simulink model "AGTF30_eng"  (R2023b)
settings: Solver=FixedStepDiscrete  StartTime=0.0  StopTime=10.0  FixedStep=0.015  RelTol=1e-3  SampleTimeConstraint=STIndependent  EnableMultiTasking=on
model workspace: external: MAT-File (data not in the file)
values from neighbouring files (symbols this model uses):
  MWS = setup_initialize(MWS,startPt,SSsolverSP)    [Setup_Simulation.m]    (also in run_AGTF30e_script.m = Setup_Simulation(inputMethod,MWS.In,filename,Mdl,SSsolverSP))
undefined symbols (not defined in the file or in its folder): stripchar_TMATS
libraries: Lib_Turbo_StaticCalc_TMATS x6, Lib_Turbo_Compressor_TMATS x3, Lib_Turbo_TurbineNPSS_TMATS x2, Lib_Turbo_Shaft_TMATS x2, Lib_Turbo_Ambient_TMATS x1, Lib_Turbo_Nozzle_TMATS x1, Lib_Turbo_NozzleVar_TMATS x1, Lib_Turbo_Burner_TMATS x1, Lib_Turbo_GearBox_TMATS x1, Lib_Turbo_Inlet_TMATS x1, Lib_Turbo_Splitter_TMATS x1, Lib_Turbo_Valve_TMATS x1
(part 2 of 2)

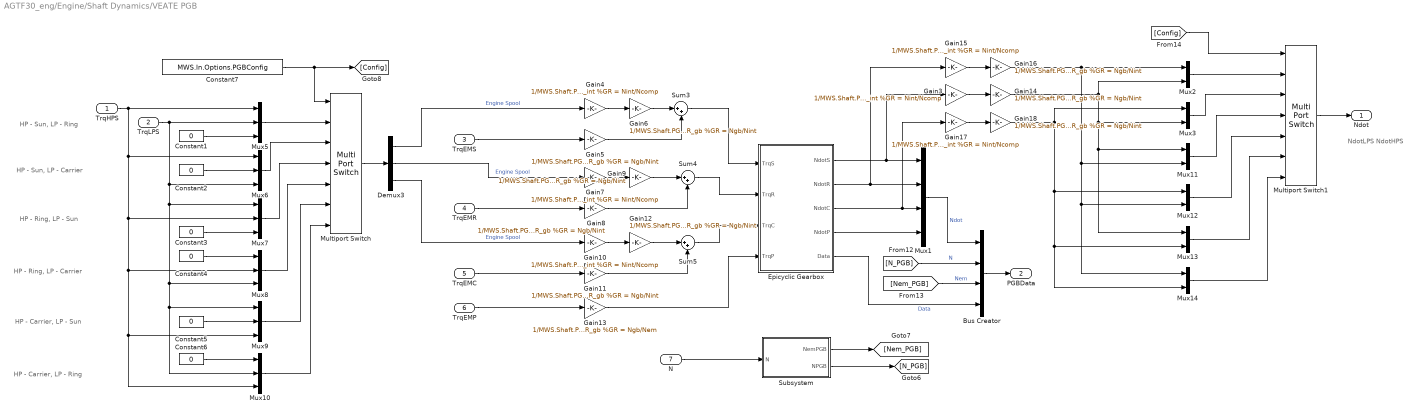
== system AGTF30_eng/Engine/Shaft Dynamics/VEATE PGB ==
  note: NdotLPS
      | NdotHPS
  note: HP - Sun, LP - Ring
  note: HP - Sun, LP - Carrier
  note: HP - Ring, LP - Sun
  note: HP - Ring, LP - Carrier
  note: HP - Carrier, LP - Sun
  note: HP - Carrier, LP - Ring
  TrqHPS : Inport
  TrqLPS : Inport  Port=2
  TrqEMS : Inport  Port=3
  TrqEMR : Inport  Port=4
  TrqEMC : Inport  Port=5
  TrqEMP : Inport  Port=6
  N : Inport  Port=7
  Bus Creator : BusCreator  Inputs=4
  Constant{1..6} (6 alike) : Constant  Value=0
  Constant7 : Constant  Value=MWS.In.Options.PGBConfig
  Demux3 : Demux  Outputs=3
  Epicyclic Gearbox : Subsystem  mask(Epicyclic Gearbox){nP_M=MWS.Shaft.PGB.Planet.nP, mP_M=MWS.Shaft.PGB.Planet.mP, rS_M=MWS.Shaft.PGB.Sun.r, rR_M=MWS.Shaft.PGB.Ring.r, JS_M=MWS.Shaft.PGB.Sun.J, JR_M=MWS.Shaft.PGB.Ring.J, JC_M=MWS.Shaft.PGB.Carrier.J, JP_M=MWS.Shaft.PGB.Planet.J}
      mask prompts: nP_M "nP_M - number of planets"; mP_M "mP_M - mass of each planet gear"; rS_M "rS_M - radius of the sun gear, ft"; rR_M "rR_M - radius of the ring gear, ft"; JS_M "JS_M - inertia of the sun gear, slug-ft^2"; JR_M "JR_M - inertia of the ring gear, slug-ft^2"; JC_M "JC_M - inertia of the carrier, slug-ft^2"; JP_M "JP_M - inertia of each planet gear, slug-ft^2"
      mask help:
      | This block models the dynamics of an epicyclic gearbox. The gearbox is made up of 3 primary components: the sun gear, the ring gear, and the carrier. The carrier is connected through axles to several planet gears that spin between the sun gear and the ring gear. Torque can be input on the sun gear (TrqS), ring gear (TrqR), carrier (TrqC), or planet gears (TrqP). The torques should be supplied in units of ft-lbf. TrqP is assumed to be applied to each planet gear. All (+) torques are prescribed to be in the same direction. This block computes the acceleration in rpm/s of each component (sun gear, ring gear, carrier, and planet gear) which can be integrated outside of the block to obtain the component speeds in rpm. The user should take care to properly intialize the speeds of the components such that the velocity of the gears at their interfaces match. In other words the following relations should be satisfied:
      |
      | rS*NC - rP*NP = rS*NS
      | rR*NC + rP*NP = rR*NR
      |
      | Given the speed of 2 of the components, the other 2 speeds can be computed. The block also provides supplemental data through the output 'Data'. This includes the forces acting at each gear interface and the effective inertia of each component. The effective inertia is defined here as the inertia experienced by the component, which accounts for the reflected inertia of the rest of the mechanical system. Also included are coefficients that describe how applying torque with each component translates to torque applied to the other components. The torque coefficients can be used together with compoent speed information to compute the impact of the gearbox relative to power injection/extraction on each component. The final parameter of the 'Data" structure is an error term that provides some evidence for confidence in the blocks calculations. The NdotErr parameter is a 4 element array that gives the difference in component accelerations calculated 2 different ways. The 4 elements of the array correspond to the sun gear, ring gear, carrier, and planet gear. For clarity, the contents of the 'Data" output are shown below:
      |
      | fsp: force in lbf acting at the sun gear and planet gear interface
      | fpr: force in lbf acting at the planet gear and ring gear interface
      | fpc: force in lbf acting at the axle connecting the planet gear to the carrier
      | JSeff: effective inertia in slug-ft^2 as seen by the sun gear
      | JReff: effective inertia in slug-ft^2 as seen by the ring gear
      | JCeff: effective inertia in slug-ft^2 as seen by the carrier
      | CTrqSR: torque coefficient relating TrqR to the torque it results in on the sun gear
      | CTrqSC: torque coefficient relating TrqC to the torque it results in on the sun gear
      | CTrqSP: torque coefficient relating TrqP to the torque it results in on the sun gear
      | CTrqRS: torque coefficient relating TrqS to the torque it results in on the ring gear
      | CTrqRC: torque coefficient relating TrqC to the torque it results in on the ring gear
      | CTrqRP: torque coefficient relating TrqP to the torque it results in on the ring gear
      | CTrqCS: torque coefficient relating TrqS to the torque it results in on the carrier
      | CTrqCR: torque coefficient relating TrqR to the torque it results in on the carrier
      | CTrqCP: torque coefficient relating TrqP to the torque it results in on the carrier
      | NdotErr: error of the component (sun gear, ring gear, carrier, planet gear) acceleratons calculated 2 separate ways.
      mask init:
      | % Planet Radius
      | rP_I = 0.5*(rR_M-rS_M);
      | % Tier 1 Simplifiers
      | lam_I = 1/(mP_M*(rS_M+rP_I));
      | zeta_I = (1/JC_M)*nP_M*(rS_M+rP_I);
      | theta_I = rP_I^2/JP_M + nP_M*rS_M^2/JS_M;
      | xi_I = rP_I^2/JP_M + nP_M*rR_M^2/JR_M;
      | % Tier 2 Simplifiers
      | phi_I = -theta_I - rP_I^2/JP_M;
      | % Tier 3 Simplifiers
      | sig_I = (1/phi_I)*(rS_M*zeta_I + theta_I*(1+zeta_I/lam_I));
      | eta_I = (1/phi_I)*(1/JC_M)*(rS_M+theta_I/lam_I);
      | alpha_I = -(rS_M/JS_M)*(1/phi_I)*(rP_I^2/JP_M+xi_I);
      | nu_I = (rP_I/JP_M)*(-(1/phi_I)*(rP_I^2/JP_M)+(-xi_I/phi_I-1));
      | % Tier 4 Simplifiers
      | gam_I = -(rP_I^2/JP_M)*(sig_I+(1+zeta_I/lam_I)) - sig_I*xi_I + rR_M*zeta_I;
      | kappa_I = sig_I + (1+zeta_I/lam_I);
      | beta_I = (rP_I^2/JP_M)*(eta_I+(1/lam_I)*(1/JC_M)) + eta_I*xi_I - rR_M/JC_M;
      | % Effective Inertias
      | JSeff_I = JS_M/(1-nP_M*rS_M*(kappa_I*alpha_I/gam_I-(1/phi_I)*rS_M/JS_M));
      | JReff_I = JR_M/(1+nP_M*(sig_I/gam_I)*(rR_M^2/JR_M));
      | JCeff_I = JC_M/(1+nP_M*(rS_M+rP_I)*beta_I/gam_I);
      | % Effective Torque Coefficients
      | CTrqSR_I = -(nP_M*rS_M*(kappa_I/gam_I)*rR_M/JR_M)/(1-nP_M*rS_M*(kappa_I*alpha_I/gam_I-(1/phi_I)*rS_M/JS_M));
      | CTrqSC_I = -(nP_M*rS_M*(kappa_I*beta_I/gam_I+eta_I+(1/lam_I)*(1/JC_M)))/(1-nP_M*rS_M*(kappa_I*alpha_I/gam_I-(1/phi_I)*rS_M/JS_M));
      | CTrqSP_I = -(nP_M*rS_M*(kappa_I*nu_I/gam_I-(1/phi_I)*(rP_I/JP_M)))/(1-nP_M*rS_M*(kappa_I*alpha_I/gam_I-(1/phi_I)*rS_M/JS_M));
      | CTrqRS_I = (nP_M*rR_M*(sig_I*alpha_I/gam_I-(1/phi_I)*rS_M/JS_M))/(1+nP_M*(sig_I/gam_I)*(rR_M^2/JR_M));
      | CTrqRC_I = (nP_M*rR_M*(sig_I*beta_I/gam_I+eta_I))/(1+nP_M*(sig_I/gam_I)*(rR_M^2/JR_M));
      | CTrqRP_I = (nP_M*rR_M*(sig_I*nu_I/gam_I-(1/phi_I)*(rP_I/JP_M)))/(1+nP_M*(sig_I/gam_I)*(rR_M^2/JR_M));
      | CTrqCS_I = (nP_M*(rS_M+rP_I)*alpha_I)/(gam_I+nP_M*(rS_M+rP_I)*beta_I);
      | CTrqCR_I = (nP_M*(rS_M+rP_I)*(rR_M/JR_M))/(gam_I+nP_M*(rS_M+rP_I)*beta_I);
      | CTrqCP_I = (nP_M*(rS_M+rP_I)*nu_I)/(gam_I+nP_M*(rS_M+rP_I)*beta_I);
  Gain10 : Gain  Gain=1/MWS.Shaft.PGB.Carrier.GR_int %GR = Nint/Ncomp
  Gain11 : Gain  Gain=1/MWS.Shaft.PGB.Carrier.GR_gb %GR = Ngb/Nint
  Gain12 : Gain  Gain=1/MWS.Shaft.PGB.Carrier.GR_gb %GR = Ngb/Nint
  Gain13 : Gain  Gain=1/MWS.Shaft.PGB.Planet.GR_gb %GR = Ngb/Nem
  Gain14 : Gain  Gain=1/MWS.Shaft.PGB.Sun.GR_gb %GR = Ngb/Nint
  Gain15 : Gain  Gain=1/MWS.Shaft.PGB.Ring.GR_int %GR = Nint/Ncomp
  Gain16 : Gain  Gain=1/MWS.Shaft.PGB.Ring.GR_gb %GR = Ngb/Nint
  Gain17 : Gain  Gain=1/MWS.Shaft.PGB.Carrier.GR_int %GR = Nint/Ncomp
  Gain18 : Gain  Gain=1/MWS.Shaft.PGB.Carrier.GR_gb %GR = Ngb/Nint
  Gain3 : Gain  Gain=1/MWS.Shaft.PGB.Sun.GR_int %GR = Nint/Ncomp
  Gain4 : Gain  Gain=1/MWS.Shaft.PGB.Sun.GR_int %GR = Nint/Ncomp
  Gain5 : Gain  Gain=1/MWS.Shaft.PGB.Sun.GR_gb %GR = Ngb/Nint
  Gain6 : Gain  Gain=1/MWS.Shaft.PGB.Sun.GR_gb %GR = Ngb/Nint
  Gain7 : Gain  Gain=1/MWS.Shaft.PGB.Ring.GR_int %GR = Nint/Ncomp
  Gain8 : Gain  Gain=1/MWS.Shaft.PGB.Ring.GR_gb %GR = Ngb/Nint
  Gain9 : Gain  Gain=1/MWS.Shaft.PGB.Ring.GR_gb %GR = Ngb/Nint
  Multiport Switch : MultiPortSwitch  Inputs=6  SaturateOnIntegerOverflow=off  InputSameDT=off
  Multiport Switch1 : MultiPortSwitch  Inputs=6  SaturateOnIntegerOverflow=off  InputSameDT=off
  Mux1 : Mux
  Mux{5..10} (6 alike) : Mux  Inputs=3
  Mux{2..3,11..14} (6 alike) : Mux  Inputs=2
  Subsystem : Subsystem
  Sum3 : Sum  Inputs=|++
  Sum4 : Sum  Inputs=|++
  Sum5 : Sum  Inputs=|++
  Ndot : Outport
  PGBData : Outport  Port=2
  wires:
  Constant5/1 -> Mux9/2
  Gain5/1 -> Sum3/2
  Gain14/1 -> Mux13/1, Mux11/1, Mux3/2, Mux2/2
  Constant3/1 -> Mux7/3
  Mux2/1 -> Multiport Switch1/2
  Mux5/1 -> Multiport Switch/2
  Gain4/1 -> Gain6/1
  Epicyclic Gearbox/2(NdotR) -> Gain15/1, Mux1/2
  Gain10/1 -> Gain12/1
  Mux14/1 -> Multiport Switch1/7
  Gain16/1 -> Mux14/1, Mux12/2, Mux11/2, Mux2/1
  Mux11/1 -> Multiport Switch1/4
  Mux13/1 -> Multiport Switch1/6
  Gain18/1 -> Mux14/2, Mux13/2, Mux12/1, Mux3/1
  Constant1/1 -> Mux5/3
  Gain12/1 -> Sum5/1
  [Config] -> Multiport Switch1/1
  Gain6/1 -> Sum3/1
  Constant7/1 -> Multiport Switch/1, [Config]
  Epicyclic Gearbox/3(NdotC) -> Gain17/1, Mux1/3
  Gain9/1 -> Sum4/1
  Mux3/1 -> Multiport Switch1/3
  Constant4/1 -> Mux8/1
  Gain15/1 -> Gain16/1
  Mux12/1 -> Multiport Switch1/5
  Sum3/1 -> Epicyclic Gearbox/1(TrqS)
  Constant6/1 -> Mux10/1
  Mux10/1 -> Multiport Switch/7
  Epicyclic Gearbox/1(NdotS) -> Gain3/1, Mux1/1
  Gain13/1 -> Epicyclic Gearbox/4(TrqP)
  Gain3/1 -> Gain14/1
  Constant2/1 -> Mux6/2
  Gain17/1 -> Gain18/1
  TrqHPS/1 -> Mux10/3, Mux9/3, Mux8/2, Mux7/2, Mux6/1, Mux5/1
  TrqEMP/1 -> Gain13/1
  Demux3/1 -> Gain4/1  "Engine Spool"
  Demux3/3 -> Gain10/1  "Engine Spool"
  Sum4/1 -> Epicyclic Gearbox/2(TrqR)
  Gain8/1 -> Sum4/2
  Mux8/1 -> Multiport Switch/5
  Multiport Switch/1 -> Demux3/1
  Gain11/1 -> Sum5/2
  Sum5/1 -> Epicyclic Gearbox/3(TrqC)
  TrqLPS/1 -> Mux6/3, Mux7/1, Mux8/3, Mux9/1, Mux10/2, Mux5/2
  Gain7/1 -> Gain9/1
  Mux7/1 -> Multiport Switch/4
  Mux6/1 -> Multiport Switch/3
  Demux3/2 -> Gain7/1  "Engine Spool"
  Mux9/1 -> Multiport Switch/6
  TrqEMC/1 -> Gain11/1
  Epicyclic Gearbox/4(NdotP) -> Mux1/4
  Mux1/1 -> Bus Creator/1  "Ndot"
  Multiport Switch1/1 -> Ndot/1
  TrqEMR/1 -> Gain8/1
  TrqEMS/1 -> Gain5/1
  Epicyclic Gearbox/5(Data) -> Bus Creator/4  "Data"
  Bus Creator/1 -> PGBData/1
  [N_PGB] -> Bus Creator/2  "N"
  [Nem_PGB] -> Bus Creator/3  "Nem"
  N/1 -> Subsystem/1(N)
  Subsystem/1(NemPGB) -> [Nem_PGB]
  Subsystem/2(NPGB) -> [N_PGB]

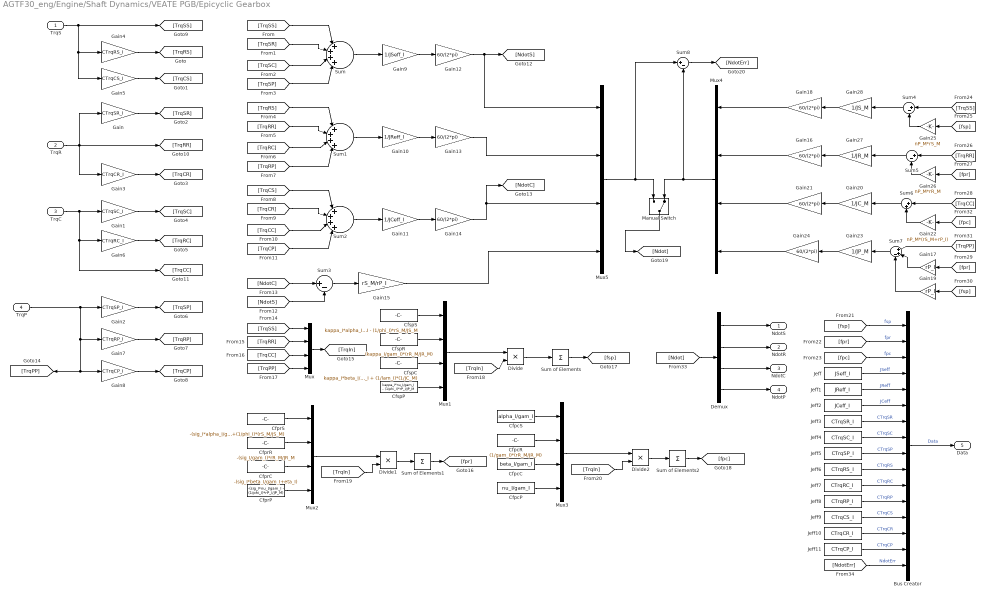
== system AGTF30_eng/Engine/Shaft Dynamics/VEATE PGB/Epicyclic Gearbox ==
  TrqS : Inport
  TrqR : Inport  Port=2
  TrqC : Inport  Port=3
  TrqP : Inport  Port=4
  Bus Creator : BusCreator  Inputs=16
  CfpcC : Constant  Value=beta_I/gam_I
  CfpcP : Constant  Value=nu_I/gam_I
  CfpcR : Constant  Value=(1/gam_I)*(rR_M/JR_M)
  CfpcS : Constant  Value=alpha_I/gam_I
  CfprC : Constant  Value=-(sig_I*beta_I/gam_I+eta_I)
  CfprP : Constant  Value=-(sig_I*nu_I/gam_I - (1/phi_I)*rP_I/JP_M)
  CfprR : Constant  Value=-(sig_I/gam_I)*rR_M/JR_M
  CfprS : Constant  Value=-(sig_I*alpha_I/gam_I)+(1/phi_I)*(rS_M/JS_M)
  CfspC : Constant  Value=kappa_I*beta_I/gam_I + eta_I + (1/lam_I)*(1/JC_M)
  CfspP : Constant  Value=kappa_I*nu_I/gam_I - (1/phi_I)*rP_I/JP_M
  CfspR : Constant  Value=(kappa_I/gam_I)*(rR_M/JR_M)
  CfspS : Constant  Value=kappa_I*alpha_I/gam_I - (1/phi_I)*rS_M/JS_M
  Demux : Demux
  Divide : Product  Inputs=**
  Divide1 : Product  Inputs=**
  Divide2 : Product  Inputs=**
  Gain : Gain  Gain=CTrqSR_I
  Gain1 : Gain  Gain=CTrqSC_I
  Gain10 : Gain  Gain=1/JReff_I
  Gain11 : Gain  Gain=1/JCeff_I
  Gain{12..14,16,18,21,24} (7 alike) : Gain  Gain=60/(2*pi)
  Gain15 : Gain  Gain=rS_M/rP_I
  Gain17 : Gain  Gain=rP_I
  Gain19 : Gain  Gain=rP_I
  Gain2 : Gain  Gain=CTrqSP_I
  Gain20 : Gain  Gain=1/JC_M
  Gain22 : Gain  Gain=nP_M*(rS_M+rP_I)
  Gain23 : Gain  Gain=1/JP_M
  Gain25 : Gain  Gain=nP_M*rS_M
  Gain26 : Gain  Gain=nP_M*rR_M
  Gain27 : Gain  Gain=1/JR_M
  Gain28 : Gain  Gain=1/JS_M
  Gain3 : Gain  Gain=CTrqCR_I
  Gain4 : Gain  Gain=CTrqRS_I
  Gain5 : Gain  Gain=CTrqCS_I
  Gain6 : Gain  Gain=CTrqRC_I
  Gain7 : Gain  Gain=CTrqRP_I
  Gain8 : Gain  Gain=CTrqCP_I
  Gain9 : Gain  Gain=1/JSeff_I
  Jeff : Constant  Value=JSeff_I
  Jeff1 : Constant  Value=JReff_I
  Jeff10 : Constant  Value=CTrqCR_I
  Jeff11 : Constant  Value=CTrqCP_I
  Jeff2 : Constant  Value=JCeff_I
  Jeff3 : Constant  Value=CTrqSR_I
  Jeff4 : Constant  Value=CTrqSC_I
  Jeff5 : Constant  Value=CTrqSP_I
  Jeff6 : Constant  Value=CTrqRS_I
  Jeff7 : Constant  Value=CTrqRC_I
  Jeff8 : Constant  Value=CTrqRP_I
  Jeff9 : Constant  Value=CTrqCS_I
  Manual Switch : ManualSwitch  CurrentSetting=0
  Mux{,1..3} (4 alike) : Mux
  Mux4 : Mux  Inputs=[1 1 1 1]
  Mux5 : Mux  Inputs=[1 1 1 1]
  Sum : Sum  Inputs=|++++|
  Sum of Elements : Sum  Inputs=+
  Sum of Elements1 : Sum  Inputs=+
  Sum of Elements2 : Sum  Inputs=+
  Sum1 : Sum  Inputs=|++++|
  Sum2 : Sum  Inputs=|++++|
  Sum{3..5,8} (4 alike) : Sum  Inputs=|+-
  Sum6 : Sum  Inputs=|++
  Sum7 : Sum  Inputs=|++-
  NdotS : Outport
  NdotR : Outport  Port=2
  NdotC : Outport  Port=3
  NdotP : Outport  Port=4
  Data : Outport  Port=5
  wires:
  TrqR/1 -> [TrqRR], Gain3/1, Gain/1
  TrqS/1 -> Gain5/1, Gain4/1, [TrqSS]
  TrqC/1 -> [TrqCC], Gain6/1, Gain1/1
  Gain4/1 -> [TrqRS]
  Gain5/1 -> [TrqCS]
  Gain/1 -> [TrqSR]
  Gain3/1 -> [TrqCR]
  Gain1/1 -> [TrqSC]
  Gain6/1 -> [TrqRC]
  Gain2/1 -> [TrqSP]
  Gain7/1 -> [TrqRP]
  Gain8/1 -> [TrqCP]
  [TrqSS] -> Sum/1
  [TrqSR] -> Sum/2
  [TrqSC] -> Sum/3
  [TrqSP] -> Sum/4
  [TrqRC] -> Sum1/3
  [TrqRP] -> Sum1/4
  [TrqRS] -> Sum1/1
  [TrqRR] -> Sum1/2
  [TrqCS] -> Sum2/1
  [TrqCP] -> Sum2/4
  [TrqCR] -> Sum2/2
  [TrqCC] -> Sum2/3
  Sum/1 -> Gain9/1
  Sum1/1 -> Gain10/1
  Sum2/1 -> Gain11/1
  Gain9/1 -> Gain12/1
  Gain10/1 -> Gain13/1
  Gain11/1 -> Gain14/1
  Gain12/1 -> Mux5/1, [NdotS]
  Gain13/1 -> Mux5/2
  Gain14/1 -> Mux5/3, [NdotC]
  [NdotC] -> Sum3/1
  [NdotS] -> Sum3/2
  Sum3/1 -> Gain15/1
  [TrqPP] -> Mux/4
  [TrqCC] -> Mux/3
  [TrqRR] -> Mux/2
  [TrqSS] -> Mux/1
  Mux/1 -> [TrqIn]
  CfspS/1 -> Mux1/1
  CfspR/1 -> Mux1/2
  CfspC/1 -> Mux1/3
  CfspP/1 -> Mux1/4
  Mux1/1 -> Divide/1
  [TrqIn] -> Divide/2
  Divide/1 -> Sum of Elements/1
  CfprC/1 -> Mux2/3
  CfprS/1 -> Mux2/1
  CfprR/1 -> Mux2/2
  CfprP/1 -> Mux2/4
  [TrqIn] -> Divide1/2
  Mux2/1 -> Divide1/1
  CfpcR/1 -> Mux3/2
  CfpcS/1 -> Mux3/1
  CfpcC/1 -> Mux3/3
  CfpcP/1 -> Mux3/4
  [TrqIn] -> Divide2/2
  Mux3/1 -> Divide2/1
  Divide1/1 -> Sum of Elements1/1
  Divide2/1 -> Sum of Elements2/1
  Sum of Elements/1 -> [fsp]
  Sum of Elements1/1 -> [fpr]
  Sum of Elements2/1 -> [fpc]
  Bus Creator/1 -> Data/1  "Data"
  [fsp] -> Bus Creator/1  "fsp"
  [fpr] -> Bus Creator/2  "fpr"
  [fpc] -> Bus Creator/3  "fpc"
  Jeff/1 -> Bus Creator/4  "JSeff"
  Jeff1/1 -> Bus Creator/5  "JReff"
  Jeff2/1 -> Bus Creator/6  "JCeff"
  Jeff3/1 -> Bus Creator/7  "CTrqSR"
  Jeff4/1 -> Bus Creator/8  "CTrqSC"
  Jeff5/1 -> Bus Creator/9  "CTrqSP"
  Jeff6/1 -> Bus Creator/10  "CTrqRS"
  Jeff7/1 -> Bus Creator/11  "CTrqRC"
  Jeff8/1 -> Bus Creator/12  "CTrqRP"
  Jeff9/1 -> Bus Creator/13  "CTrqCS"
  Jeff10/1 -> Bus Creator/14  "CTrqCR"
  Jeff11/1 -> Bus Creator/15  "CTrqCP"
  TrqP/1 -> Gain2/1, Gain8/1, [TrqPP], Gain7/1
  Gain15/1 -> Mux5/4
  Gain23/1 -> Gain24/1
  Sum4/1 -> Gain28/1
  Gain25/1 -> Sum4/2
  Gain28/1 -> Gain18/1
  [fsp] -> Gain19/1
  [TrqSS] -> Sum4/1
  Sum6/1 -> Gain20/1
  [fpc] -> Gain22/1
  Sum7/1 -> Gain23/1
  [fpr] -> Gain17/1
  Gain17/1 -> Sum7/2
  [fpr] -> Gain26/1
  Gain22/1 -> Sum6/2
  Gain26/1 -> Sum5/2
  Gain27/1 -> Gain16/1
  Sum5/1 -> Gain27/1
  [TrqPP] -> Sum7/1
  Gain20/1 -> Gain21/1
  [TrqRR] -> Sum5/1
  [TrqCC] -> Sum6/1
  [fsp] -> Gain25/1
  Gain18/1 -> Mux4/1
  Sum8/1 -> [NdotErr]
  [NdotErr] -> Bus Creator/16  "NdotErr"
  Gain19/1 -> Sum7/3
  Gain24/1 -> Mux4/4
  Gain21/1 -> Mux4/3
  Gain16/1 -> Mux4/2
  Mux5/1 -> Sum8/1, Manual Switch/1
  Mux4/1 -> Manual Switch/2, Sum8/2
  Manual Switch/1 -> [Ndot]
  [Ndot] -> Demux/1
  Demux/4 -> NdotP/1
  Demux/3 -> NdotC/1
  Demux/2 -> NdotR/1
  Demux/1 -> NdotS/1

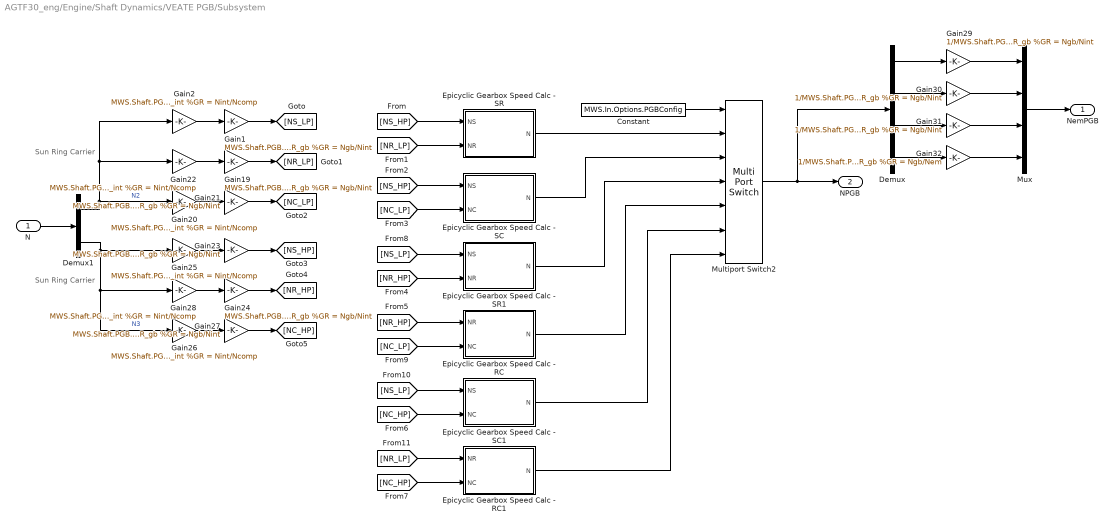
== system AGTF30_eng/Engine/Shaft Dynamics/VEATE PGB/Subsystem ==
  note: Sun
      | Ring
      | Carrier
  note: Sun
      | Ring
      | Carrier
  N : Inport
  Constant : Constant  Value=MWS.In.Options.PGBConfig
  Demux : Demux
  Demux1 : Demux  Outputs=2
  Epicyclic Gearbox Speed Calc - RC : Subsystem  mask(Epicyclic Gearbox Speed Calc - SC){rS_M=MWS.Shaft.PGB.Sun.r, rR_M=MWS.Shaft.PGB.Ring.r}
      mask prompts: rS_M "rS_M - Sun gear radius, ft"; rR_M "rR_M - Ring gear radius, ft"
      mask help: This block outputs the rotational speeds of all 4 epicyclic gearbox components (sun, ring, carrier, planets) given the speeds of the sun gear and carrier. Units are consistent with input units.
      mask init:
      | rP_I = 0.5*(rR_M-rS_M);
  Epicyclic Gearbox Speed Calc - RC1 : Subsystem  mask(Epicyclic Gearbox Speed Calc - SC){rS_M=MWS.Shaft.PGB.Sun.r, rR_M=MWS.Shaft.PGB.Ring.r}
      mask prompts: rS_M "rS_M - Sun gear radius, ft"; rR_M "rR_M - Ring gear radius, ft"
      mask help: This block outputs the rotational speeds of all 4 epicyclic gearbox components (sun, ring, carrier, planets) given the speeds of the sun gear and carrier. Units are consistent with input units.
      mask init:
      | rP_I = 0.5*(rR_M-rS_M);
  Epicyclic Gearbox Speed Calc - SC : Subsystem  mask(Epicyclic Gearbox Speed Calc - SC){rS_M=MWS.Shaft.PGB.Sun.r, rR_M=MWS.Shaft.PGB.Ring.r}
      mask prompts: rS_M "rS_M - Sun gear radius, ft"; rR_M "rR_M - Ring gear radius, ft"
      mask help: This block outputs the rotational speeds of all 4 epicyclic gearbox components (sun, ring, carrier, planets) given the speeds of the sun gear and carrier. Units are consistent with input units.
      mask init:
      | rP_I = 0.5*(rR_M-rS_M);
  Epicyclic Gearbox Speed Calc - SC1 : Subsystem  mask(Epicyclic Gearbox Speed Calc - SC){rS_M=MWS.Shaft.PGB.Sun.r, rR_M=MWS.Shaft.PGB.Ring.r}
      mask prompts: rS_M "rS_M - Sun gear radius, ft"; rR_M "rR_M - Ring gear radius, ft"
      mask help: This block outputs the rotational speeds of all 4 epicyclic gearbox components (sun, ring, carrier, planets) given the speeds of the sun gear and carrier. Units are consistent with input units.
      mask init:
      | rP_I = 0.5*(rR_M-rS_M);
  Epicyclic Gearbox Speed Calc - SR : Subsystem  mask(Epicyclic Gearbox Speed Calc - SR){rS_M=MWS.Shaft.PGB.Sun.r, rR_M=MWS.Shaft.PGB.Ring.r}
      mask prompts: rS_M "rS_M - Radius of the sun gear, ft"; rR_M "rR_M - Radius of the ring gear, ft"
      mask help: This block outputs the rotational speeds of all 4 epicyclic gearbox components (sun, ring, carrier, planets) given the speeds of the sun gear and ring gear. Units are consistent with input units.
      mask init:
      | rP_I = 0.5*(rR_M-rS_M);
  Epicyclic Gearbox Speed Calc - SR1 : Subsystem  mask(Epicyclic Gearbox Speed Calc - SR){rS_M=MWS.Shaft.PGB.Sun.r, rR_M=MWS.Shaft.PGB.Ring.r}
      mask prompts: rS_M "rS_M - Radius of the sun gear, ft"; rR_M "rR_M - Radius of the ring gear, ft"
      mask help: This block outputs the rotational speeds of all 4 epicyclic gearbox components (sun, ring, carrier, planets) given the speeds of the sun gear and ring gear. Units are consistent with input units.
      mask init:
      | rP_I = 0.5*(rR_M-rS_M);
  Gain1 : Gain  Gain=MWS.Shaft.PGB.Sun.GR_gb %GR = Ngb/Nint
  Gain19 : Gain  Gain=MWS.Shaft.PGB.Ring.GR_gb %GR = Ngb/Nint
  Gain2 : Gain  Gain=MWS.Shaft.PGB.Sun.GR_int %GR = Nint/Ncomp
  Gain20 : Gain  Gain=MWS.Shaft.PGB.Carrier.GR_int %GR = Nint/Ncomp
  Gain21 : Gain  Gain=MWS.Shaft.PGB.Carrier.GR_gb %GR = Ngb/Nint
  Gain22 : Gain  Gain=MWS.Shaft.PGB.Ring.GR_int %GR = Nint/Ncomp
  Gain23 : Gain  Gain=MWS.Shaft.PGB.Sun.GR_gb %GR = Ngb/Nint
  Gain24 : Gain  Gain=MWS.Shaft.PGB.Ring.GR_gb %GR = Ngb/Nint
  Gain25 : Gain  Gain=MWS.Shaft.PGB.Sun.GR_int %GR = Nint/Ncomp
  Gain26 : Gain  Gain=MWS.Shaft.PGB.Carrier.GR_int %GR = Nint/Ncomp
  Gain27 : Gain  Gain=MWS.Shaft.PGB.Carrier.GR_gb %GR = Ngb/Nint
  Gain28 : Gain  Gain=MWS.Shaft.PGB.Ring.GR_int %GR = Nint/Ncomp
  Gain29 : Gain  Gain=1/MWS.Shaft.PGB.Sun.GR_gb %GR = Ngb/Nint
  Gain30 : Gain  Gain=1/MWS.Shaft.PGB.Ring.GR_gb %GR = Ngb/Nint
  Gain31 : Gain  Gain=1/MWS.Shaft.PGB.Carrier.GR_gb %GR = Ngb/Nint
  Gain32 : Gain  Gain=1/MWS.Shaft.PGB.Planet.GR_gb %GR = Ngb/Nem
  Multiport Switch2 : MultiPortSwitch  Inputs=6  SaturateOnIntegerOverflow=off  InputSameDT=off
  Mux : Mux
  NemPGB : Outport
  NPGB : Outport  Port=2
  wires:
  Demux1/1 -> Gain20/1, Gain22/1, Gain2/1  "N2"
  Gain27/1 -> [NC_HP]
  Epicyclic Gearbox Speed Calc - RC1/1(N) -> Multiport Switch2/7
  Epicyclic Gearbox Speed Calc - SR1/1(N) -> Multiport Switch2/4
  Gain31/1 -> Mux/3
  Demux/3 -> Gain31/1
  Gain22/1 -> Gain19/1
  [NS_LP] -> Epicyclic Gearbox Speed Calc - SR1/1(NS)
  Gain30/1 -> Mux/2
  [NR_LP] -> Epicyclic Gearbox Speed Calc - RC1/1(NR)
  Demux/2 -> Gain30/1
  N/1 -> Demux1/1
  Gain20/1 -> Gain21/1
  Gain28/1 -> Gain24/1
  [NC_LP] -> Epicyclic Gearbox Speed Calc - SC/2(NC)
  Gain2/1 -> Gain1/1
  [NS_HP] -> Epicyclic Gearbox Speed Calc - SC/1(NS)
  Multiport Switch2/1 -> NPGB/1, Demux/1
  [NR_LP] -> Epicyclic Gearbox Speed Calc - SR/2(NR)
  Demux/1 -> Gain29/1
  Gain24/1 -> [NR_HP]
  Gain32/1 -> Mux/4
  Gain29/1 -> Mux/1
  [NR_HP] -> Epicyclic Gearbox Speed Calc - RC/1(NR)
  Demux/4 -> Gain32/1
  Demux1/2 -> Gain26/1, Gain28/1, Gain25/1  "N3"
  Gain26/1 -> Gain27/1
  Gain25/1 -> Gain23/1
  Gain1/1 -> [NS_LP]
  Epicyclic Gearbox Speed Calc - SC/1(N) -> Multiport Switch2/3
  [NS_HP] -> Epicyclic Gearbox Speed Calc - SR/1(NS)
  Gain19/1 -> [NR_LP]
  Gain21/1 -> [NC_LP]
  Gain23/1 -> [NS_HP]
  Epicyclic Gearbox Speed Calc - SR/1(N) -> Multiport Switch2/2
  [NC_HP] -> Epicyclic Gearbox Speed Calc - SC1/2(NC)
  [NC_HP] -> Epicyclic Gearbox Speed Calc - RC1/2(NC)
  [NS_LP] -> Epicyclic Gearbox Speed Calc - SC1/1(NS)
  Epicyclic Gearbox Speed Calc - RC/1(N) -> Multiport Switch2/5
  Constant/1 -> Multiport Switch2/1
  [NR_HP] -> Epicyclic Gearbox Speed Calc - SR1/2(NR)
  [NC_LP] -> Epicyclic Gearbox Speed Calc - RC/2(NC)
  Epicyclic Gearbox Speed Calc - SC1/1(N) -> Multiport Switch2/6
  Mux/1 -> NemPGB/1

== system AGTF30_eng/Engine/Shaft Dynamics/VEATE PGB/Subsystem/Epicyclic Gearbox Speed Calc - RC ==
  NR : Inport
  NC : Inport  Port=2
  Gain1 : Gain  Gain=rP_I
  Gain2 : Gain  Gain=rS_M
  Gain30 : Gain  Gain=rR_M/rP_I
  Gain31 : Gain  Gain=1/rS_M
  Mux4 : Mux
  Sum : Sum  Inputs=|+-
  Sum2 : Sum  Inputs=|+-
  N : Outport
  wires:
  NC/1 -> Gain2/1, Mux4/3, Sum/2  "NC"
  NR/1 -> Mux4/2, Sum/1  "NR"
  Mux4/1 -> N/1
  Sum/1 -> Gain30/1
  Gain30/1 -> Mux4/4, Gain1/1  "NP"
  Gain1/1 -> Sum2/2
  Gain2/1 -> Sum2/1
  Sum2/1 -> Gain31/1
  Gain31/1 -> Mux4/1  "NS"

== system AGTF30_eng/Engine/Shaft Dynamics/VEATE PGB/Subsystem/Epicyclic Gearbox Speed Calc - RC1 ==
  NR : Inport
  NC : Inport  Port=2
  Gain1 : Gain  Gain=rP_I
  Gain2 : Gain  Gain=rS_M
  Gain30 : Gain  Gain=rR_M/rP_I
  Gain31 : Gain  Gain=1/rS_M
  Mux4 : Mux
  Sum : Sum  Inputs=|+-
  Sum2 : Sum  Inputs=|+-
  N : Outport
  wires:
  Gain31/1 -> Mux4/1  "NS"
  Sum2/1 -> Gain31/1
  Gain2/1 -> Sum2/1
  Gain1/1 -> Sum2/2
  Gain30/1 -> Gain1/1, Mux4/4  "NP"
  Sum/1 -> Gain30/1
  Mux4/1 -> N/1
  NR/1 -> Sum/1, Mux4/2  "NR"
  NC/1 -> Sum/2, Mux4/3, Gain2/1  "NC"

== system AGTF30_eng/Engine/Shaft Dynamics/VEATE PGB/Subsystem/Epicyclic Gearbox Speed Calc - SC ==
  NS : Inport
  NC : Inport  Port=2
  Gain1 : Gain  Gain=rP_I
  Gain2 : Gain  Gain=rR_M
  Gain30 : Gain  Gain=rS_M/rP_I
  Gain31 : Gain  Gain=1/rR_M
  Mux4 : Mux
  Sum : Sum  Inputs=|-+
  Sum1 : Sum  Inputs=|++
  N : Outport
  wires:
  Mux4/1 -> N/1
  Gain31/1 -> Mux4/2  "NR"
  Gain30/1 -> Mux4/4, Gain1/1  "NP"
  NS/1 -> Sum/1, Mux4/1  "NS"
  Sum1/1 -> Gain31/1
  NC/1 -> Gain2/1, Mux4/3, Sum/2  "NC"
  Sum/1 -> Gain30/1
  Gain1/1 -> Sum1/1
  Gain2/1 -> Sum1/2

== system AGTF30_eng/Engine/Shaft Dynamics/VEATE PGB/Subsystem/Epicyclic Gearbox Speed Calc - SC1 ==
  NS : Inport
  NC : Inport  Port=2
  Gain1 : Gain  Gain=rP_I
  Gain2 : Gain  Gain=rR_M
  Gain30 : Gain  Gain=rS_M/rP_I
  Gain31 : Gain  Gain=1/rR_M
  Mux4 : Mux
  Sum : Sum  Inputs=|-+
  Sum1 : Sum  Inputs=|++
  N : Outport
  wires:
  Gain2/1 -> Sum1/2
  Gain1/1 -> Sum1/1
  Sum/1 -> Gain30/1
  NC/1 -> Sum/2, Mux4/3, Gain2/1  "NC"
  Sum1/1 -> Gain31/1
  NS/1 -> Mux4/1, Sum/1  "NS"
  Gain30/1 -> Gain1/1, Mux4/4  "NP"
  Gain31/1 -> Mux4/2  "NR"
  Mux4/1 -> N/1

== system AGTF30_eng/Engine/Shaft Dynamics/VEATE PGB/Subsystem/Epicyclic Gearbox Speed Calc - SR ==
  NS : Inport
  NR : Inport  Port=2
  Gain : Gain  Gain=rS_M
  Gain29 : Gain  Gain=rR_M
  Gain30 : Gain  Gain=1/(rS_M+rR_M)
  Gain31 : Gain  Gain=rS_M/rP_I
  Mux4 : Mux
  Sum : Sum  Inputs=|++
  Sum1 : Sum  Inputs=-+|
  N : Outport
  wires:
  NS/1 -> Mux4/1, Sum1/1, Gain/1
  Sum/1 -> Gain30/1
  Gain29/1 -> Sum/2
  NR/1 -> Mux4/2, Gain29/1
  Sum1/1 -> Gain31/1
  Gain/1 -> Sum/1
  Gain30/1 -> Mux4/3, Sum1/2  "NC"
  Gain31/1 -> Mux4/4  "NP"
  Mux4/1 -> N/1

== system AGTF30_eng/Engine/Shaft Dynamics/VEATE PGB/Subsystem/Epicyclic Gearbox Speed Calc - SR1 ==
  NS : Inport
  NR : Inport  Port=2
  Gain : Gain  Gain=rS_M
  Gain29 : Gain  Gain=rR_M
  Gain30 : Gain  Gain=1/(rS_M+rR_M)
  Gain31 : Gain  Gain=rS_M/rP_I
  Mux4 : Mux
  Sum : Sum  Inputs=|++
  Sum1 : Sum  Inputs=-+|
  N : Outport
  wires:
  Mux4/1 -> N/1
  Gain31/1 -> Mux4/4  "NP"
  Gain30/1 -> Mux4/3, Sum1/2  "NC"
  Gain/1 -> Sum/1
  Sum1/1 -> Gain31/1
  NR/1 -> Gain29/1, Mux4/2
  Gain29/1 -> Sum/2
  Sum/1 -> Gain30/1
  NS/1 -> Gain/1, Sum1/1, Mux4/1
